simulink model "Mission_B"  (R2019b)
settings: Solver=VariableStepAuto  StartTime=0.0  StopTime=10.0  RelTol=1e-3
settings Model: Creator=visha  LastModifiedBy=visha
settings OptimizationCC: DefaultParameterBehavior=Inlined

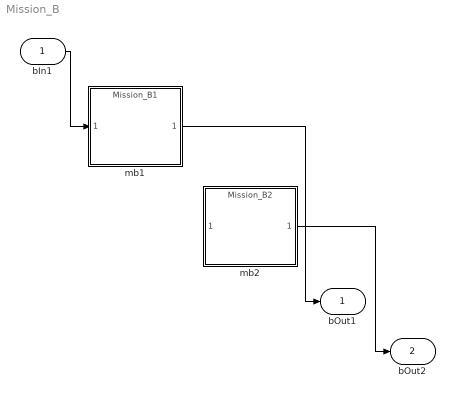
== system Mission_B ==
  bIn1 : Inport  OutDataTypeStr=int32
  mb1 : ModelReference  ModelNameDialog=Mission_B1  SimulationMode=Normal  ModelReferenceVersion=1.1
  mb2 : ModelReference  ModelNameDialog=Mission_B2  SimulationMode=Normal  ModelReferenceVersion=1.1
  bOut1 : Outport  OutDataTypeStr=int32
  bOut2 : Outport  Port=2  OutDataTypeStr=int32
  wires:
  bIn1/1 -> mb1/1
  mb1/1 -> bOut1/1
  mb2/1 -> bOut2/1
